simulink model "MACHINECC"  (R2014a)
settings: Solver=ode45  StartTime=0.0  StopTime=30.0  MaxStep=1e-3  RelTol=1e-3
undefined symbols (not defined in the file or in its folder): f, J, K, Kpi, Kpi2, L, R, Ti, Ti2
settings Model: Creator=ciottopinton_gus  LastModifiedBy=gciotto
settings DebuggingCC: UnderspecifiedInitializationDetection=Classic  StateNameClashWarn=warning

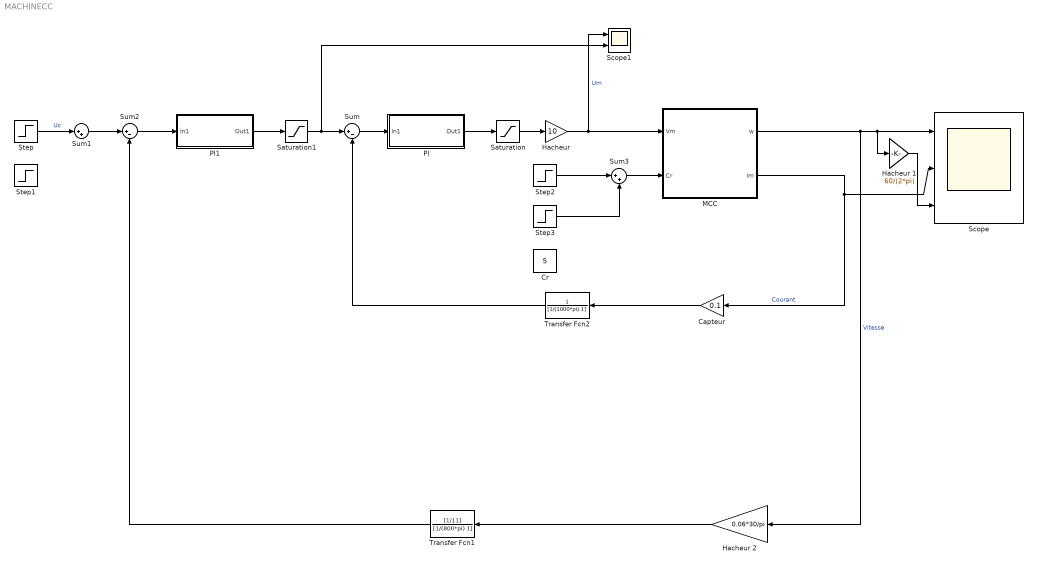
== system MACHINECC ==
  Capteur : Gain  Gain=0.1
  Cr : Constant  Value=5
  "Hacheur " : Gain  Gain=10
  Hacheur 1 : Gain  Gain=60/(2*pi)
  Hacheur 2 : Gain  Gain=0.06*30/pi
  MCC : Subsystem
  PI : Subsystem
  PI1 : Subsystem
  Saturation : Saturate  UpperLimit=9  LowerLimit=-9
  Saturation1 : Saturate  UpperLimit=4  LowerLimit=-4
  Scope : Scope  NumInputPorts=3
      settings: YMin=-5~-5~-5  YMax=5~5~5
  Scope1 : Scope  NumInputPorts=2
      settings: YMin=-5~-5  YMax=5~5
  Step : Step  Time=0  After=0.06/11*800  SampleTime=0
  Step1 : Step  Time=3  After=-4  SampleTime=0
  Step2 : Step  Time=5  After=15  SampleTime=0
  Step3 : Step  Time=15  After=-10  SampleTime=0
  Sum : Sum  Inputs=|+-
  Sum1 : Sum  Inputs=|++
  Sum2 : Sum  Inputs=|+-
  Sum3 : Sum  Inputs=|++
  Transfer Fcn1 : TransferFcn  Numerator=[1/11]  Denominator=[1/(800*pi) 1]
  Transfer Fcn2 : TransferFcn  Denominator=[1/(1000*pi) 1]
  wires:
  "Hacheur "/1 -> Scope1/1, MCC/1("Vm ")  "Um"
  MCC/2(Im) -> Capteur/1, Scope/2  "Courant"
  Capteur/1 -> Transfer Fcn2/1
  Transfer Fcn2/1 -> Sum/2
  Saturation/1 -> "Hacheur "/1
  Sum/1 -> PI/1(In1)
  PI/1(Out1) -> Saturation/1
  Step/1 -> Sum1/1  "Uc"
  MCC/1(w) -> Hacheur 2/1, Scope/1, Hacheur 1/1  "Vitesse"
  Hacheur 2/1 -> Transfer Fcn1/1
  Transfer Fcn1/1 -> Sum2/2
  Sum1/1 -> Sum2/1
  Sum2/1 -> PI1/1(In1)
  PI1/1(Out1) -> Saturation1/1
  Saturation1/1 -> Scope1/2, Sum/1
  Hacheur 1/1 -> Scope/3
  Sum3/1 -> MCC/2("Cr ")
  Step3/1 -> Sum3/2
  Step2/1 -> Sum3/1

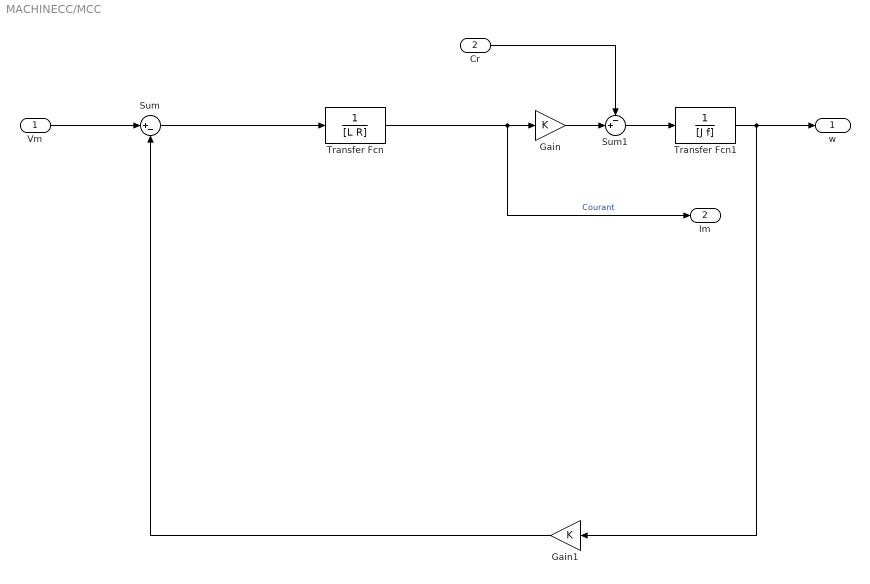
== system MACHINECC/MCC ==
  "Vm " : Inport
  "Cr " : Inport  Port=2
  Gain : Gain  Gain=K
  Gain1 : Gain  Gain=K
  Sum : Sum  Inputs=|+-
  Sum1 : Sum  Inputs=-+|
  Transfer Fcn : TransferFcn  Denominator=[L R]
  Transfer Fcn1 : TransferFcn  Denominator=[J f]
  w : Outport
  Im : Outport  Port=2
  wires:
  "Vm "/1 -> Sum/1
  Gain/1 -> Sum1/2
  "Cr "/1 -> Sum1/1
  Sum1/1 -> Transfer Fcn1/1
  Transfer Fcn1/1 -> Gain1/1, w/1
  Gain1/1 -> Sum/2
  Transfer Fcn/1 -> Im/1, Gain/1  "Courant"
  Sum/1 -> Transfer Fcn/1

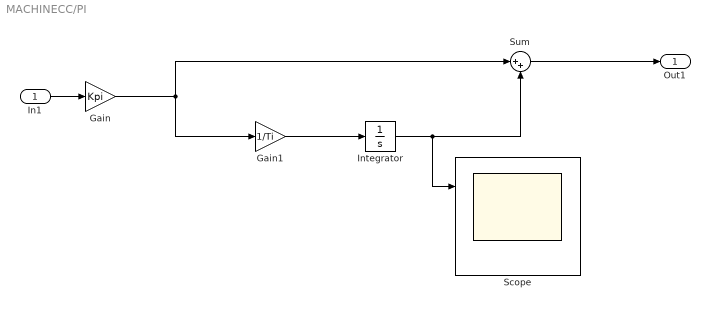
== system MACHINECC/PI ==
  In1 : Inport
  Gain : Gain  Gain=Kpi
  Gain1 : Gain  Gain=1/Ti
  Integrator : Integrator  LimitOutput=on  UpperSaturationLimit=9  LowerSaturationLimit=-9
  Scope : Scope  NumInputPorts=2
      settings: YMin=-5~-5  YMax=5~5  SaveName=ScopeData2
  Sum : Sum  Inputs=|++
  Out1 : Outport
  wires:
  In1/1 -> Gain/1
  Gain/1 -> Sum/1, Gain1/1
  Gain1/1 -> Integrator/1
  Integrator/1 -> Scope/1, Sum/2
  Sum/1 -> Out1/1

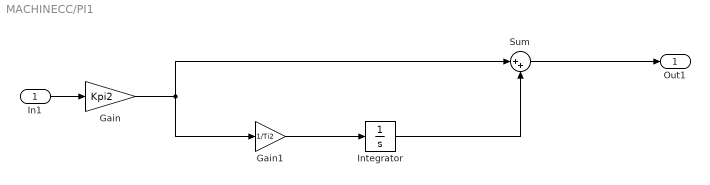
== system MACHINECC/PI1 ==
  In1 : Inport
  Gain : Gain  Gain=Kpi2
  Gain1 : Gain  Gain=1/Ti2
  Integrator : Integrator
  Sum : Sum  Inputs=|++
  Out1 : Outport
  wires:
  In1/1 -> Gain/1
  Gain/1 -> Sum/1, Gain1/1
  Gain1/1 -> Integrator/1
  Integrator/1 -> Sum/2
  Sum/1 -> Out1/1
